simulink model "controllo_giunti_R2020b"  (R2020b)
settings: Solver=FixedStepAuto  StartTime=0.0  StopTime=1  FixedStep=0.001  RelTol=1e-3
undefined symbols (not defined in the file or in its folder): f_G1, f_G2, f_G3, f_M11, f_M12, f_M13, f_M21, f_M22, f_M23, f_M31, f_M32, f_M33, f_V1, f_V2, f_V3
libraries: robotcorelib x1
settings Model: Creator=frasi  LastModifiedBy=frasi

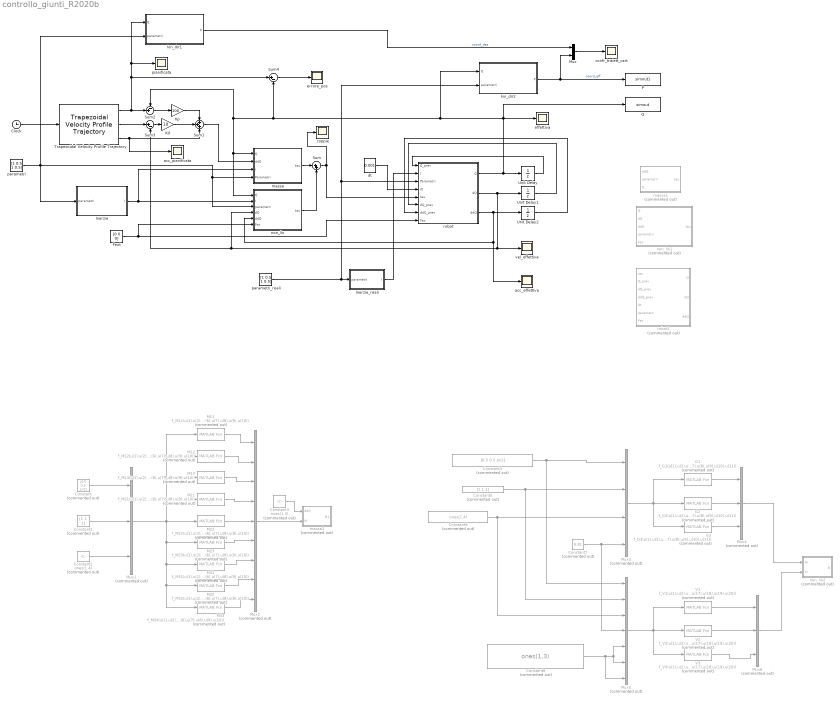
== system controllo_giunti_R2020b ==
  Clock : Clock
  Constant : Constant  Commented=on  Value=[0.5 0.5 pi/2]
  Constant1 : Constant  Commented=on  Value=[1 1 1]
  Constant2 : Constant  Commented=on  Value=ones(1,4)
  Constant3 : Constant  Commented=on  Value=ones(1,3)
  Constant4 : Constant  Commented=on  Value=[0.5 0.5 pi/2]
  Constant5 : Constant  Commented=on  Value=[1 1 1]
  Constant6 : Constant  Commented=on  Value=ones(1,4)
  Constant7 : Constant  Commented=on  Value=9.81
  Constant8 : Constant  Commented=on  Value=ones(1,3)
  Fext : Constant  Value=[0 0 0]
  G1 : MATLABFcn  Commented=on  MATLABFcn=f_G1(u(1),u(2),u(3),u(4),u(5),u(6),u(7),u(8),u(9),u(10),u(11))
  G2 : MATLABFcn  Commented=on  MATLABFcn=f_G2(u(1),u(2),u(3),u(4),u(5),u(6),u(7),u(8),u(9),u(10),u(11))
  G3 : MATLABFcn  Commented=on  MATLABFcn=f_G3(u(1),u(2),u(3),u(4),u(5),u(6),u(7),u(8),u(9),u(10),u(11))
  Inerzie : MATLAB Function  TreatAsAtomicUnit=on
  Inerzie_reali : MATLAB Function  TreatAsAtomicUnit=on
  Kd : Gain  Gain=10
  Kp : Gain  Gain=100
  M11 : MATLABFcn  Commented=on  MATLABFcn=f_M11(u(1),u(2),u(3),u(4),u(5),u(6),u(7),u(8),u(9),u(10))
  M12 : MATLABFcn  Commented=on  MATLABFcn=f_M12(u(1),u(2),u(3),u(4),u(5),u(6),u(7),u(8),u(9),u(10))
  M13 : MATLABFcn  Commented=on  MATLABFcn=f_M13(u(1),u(2),u(3),u(4),u(5),u(6),u(7),u(8),u(9),u(10))
  M21 : MATLABFcn  Commented=on  MATLABFcn=f_M21(u(1),u(2),u(3),u(4),u(5),u(6),u(7),u(8),u(9),u(10))
  M22 : MATLABFcn  Commented=on  MATLABFcn=f_M22(u(1),u(2),u(3),u(4),u(5),u(6),u(7),u(8),u(9),u(10))
  M23 : MATLABFcn  Commented=on  MATLABFcn=f_M23(u(1),u(2),u(3),u(4),u(5),u(6),u(7),u(8),u(9),u(10))
  M31 : MATLABFcn  Commented=on  MATLABFcn=f_M31(u(1),u(2),u(3),u(4),u(5),u(6),u(7),u(8),u(9),u(10))
  M32 : MATLABFcn  Commented=on  MATLABFcn=f_M32(u(1),u(2),u(3),u(4),u(5),u(6),u(7),u(8),u(9),u(10))
  M33 : MATLABFcn  Commented=on  MATLABFcn=f_M33(u(1),u(2),u(3),u(4),u(5),u(6),u(7),u(8),u(9),u(10))
  Mux : Mux  Inputs=2
  Mux1 : Mux  Commented=on  Inputs=3
  Mux2 : Mux  Commented=on  Inputs=9
  Mux3 : Mux  Commented=on
  Mux4 : Mux  Commented=on  Inputs=3
  Mux5 : Mux  Commented=on  Inputs=7
  Mux6 : Mux  Commented=on  Inputs=3
  P : ToWorkspace  VariableName=simout1  SaveFormat=Timeseries  SampleTime=-1
  Q : ToWorkspace  VariableName=simout  SaveFormat=Timeseries  SampleTime=-1
  Sum : Sum  Inputs=|++
  Sum1 : Sum  Inputs=+++
  Sum2 : Sum  Inputs=-+|
  Sum3 : Sum  Inputs=|+-
  Sum4 : Sum  Inputs=|+-
  Trapezoidal Velocity Profile Trajectory : robotcorelib/Trapezoidal Velocity Profile Trajectory  WaypointSource=Internal  Waypoints=[0.5 0.7; 0.7 0.5; pi/4 pi/3]  NumParams=1  Parameter1=End Time  Parameter2=End Time  ParameterSource=Internal  PeakVelocity=[ 2; 2 ]  Acceleration=[ 1; 2 ]  EndTime=[ 1; 1 ;1]  AccelTime=[ 1; 2 ]  SimulateUsing=Interpreted execution
      settings: SourceProductBaseCode=NV,RO,RR,UV
  Unit Delay : UnitDelay  InitialCondition=[0.5 0.7 pi/4]  SampleTime=-1  HasFrameUpgradeWarning=on
  Unit Delay1 : UnitDelay  InitialCondition=[0 0 0]  SampleTime=-1  HasFrameUpgradeWarning=on
  Unit Delay2 : UnitDelay  InitialCondition=[0 0 0]  SampleTime=-1  HasFrameUpgradeWarning=on
  V1 : MATLABFcn  Commented=on  MATLABFcn=f_V1(u(1),u(2),u(3),u(4),u(5),u(6),u(7),u(8),u(9),u(10),u(11),u(12),u(13),u(14),u(15),u(16),u(17),u(18),u(19),u(20))
  V2 : MATLABFcn  Commented=on  MATLABFcn=f_V2(u(1),u(2),u(3),u(4),u(5),u(6),u(7),u(8),u(9),u(10),u(11),u(12),u(13),u(14),u(15),u(16),u(17),u(18),u(19),u(20))
  V3 : MATLABFcn  Commented=on  MATLABFcn=f_V3(u(1),u(2),u(3),u(4),u(5),u(6),u(7),u(8),u(9),u(10),u(11),u(12),u(13),u(14),u(15),u(16),u(17),u(18),u(19),u(20))
  acc_effettiva : Scope
  acc_pianificata : Scope
  confr_traiett_cart : Scope
  coppie : Scope
  dt : Constant  Value=0.001
  effettiva : Scope
  errore_pos : Scope
  kin_dir1 : MATLAB Function  TreatAsAtomicUnit=on
  kin_dir2 : MATLAB Function  TreatAsAtomicUnit=on
  massa : Subsystem
  massa1 : MATLAB Function  Commented=on  TreatAsAtomicUnit=on
  massa2 : MATLAB Function  Commented=on  TreatAsAtomicUnit=on
  non_lin : Subsystem
  non_lin1 : MATLAB Function  Commented=on  TreatAsAtomicUnit=on
  non_lin2 : MATLAB Function  Commented=on  TreatAsAtomicUnit=on
  parametri : Constant  Value=[1 0.5 1 0.5]
  parametri_reali : Constant  Value=[1 0.5 1 0.5]
  pianificata : Scope
  robot : Subsystem
  robot1 : MATLAB Function  Commented=on  TreatAsAtomicUnit=on
  vel_effettiva : Scope
  wires:
  Clock/1 -> Trapezoidal Velocity Profile Trajectory/1
  parametri/1 -> Inerzie/1(parametri), kin_dir1/2(parametri), non_lin/3(parametri), massa/4(Parametri)
  massa/1(tau) -> Sum/1
  dt/1 -> robot/4(dt)
  robot/1(Q) -> Q/1, Sum4/2, Sum2/1, non_lin/1(Q), massa/1(Q), kin_dir2/1(Q), effettiva/1, Unit Delay/1
  robot/2(dQ) -> Unit Delay1/1, non_lin/4(dQ), Sum3/2, vel_effettiva/1
  Unit Delay/1 -> robot/1(Q_prev)
  Unit Delay1/1 -> robot/6(dQ_prev)
  Sum/1 -> robot/5(tau), coppie/1
  Trapezoidal Velocity Profile Trajectory/2 -> Sum3/1
  Sum2/1 -> Kp/1
  Sum3/1 -> Kd/1
  Kp/1 -> Sum1/1
  Kd/1 -> Sum1/2
  Trapezoidal Velocity Profile Trajectory/3 -> acc_pianificata/1, Sum1/3
  non_lin/1(tau) -> Sum/2
  Trapezoidal Velocity Profile Trajectory/1 -> Sum4/1, kin_dir1/1(Q), pianificata/1, Sum2/2
  robot/3(ddQ) -> Unit Delay2/1, acc_effettiva/1, non_lin/5(ddQ)
  parametri_reali/1 -> robot/3(Parametri), kin_dir2/2(parametri), Inerzie_reali/1(parametri)
  Sum4/1 -> errore_pos/1
  kin_dir1/1(P) -> Mux/1  "coord_des"
  kin_dir2/1(P) -> P/1, Mux/2  "coord_eff"
  Mux/1 -> confr_traiett_cart/1
  Fext/1 -> robot/8(Fex), non_lin/6(Fex)
  Sum1/1 -> massa/2(ddQ)
  Inerzie/1(I) -> massa/3(I), non_lin/2(I)
  Unit Delay2/1 -> robot/7(ddQ_prev)
  Inerzie_reali/1(I) -> robot/2(I)
  Constant2/1 -> Mux1/3
  Constant1/1 -> Mux1/2
  Constant3/1 -> massa2/1(ddQ)
  Mux1/1 -> M13/1, M12/1, M11/1, M21/1, M31/1, M32/1, M33/1, M23/1, M22/1
  M23/1 -> Mux2/6
  M33/1 -> Mux2/9
  M22/1 -> Mux2/5
  Mux2/1 -> massa2/2(M)
  M11/1 -> Mux2/1
  M32/1 -> Mux2/8
  M21/1 -> Mux2/4
  M31/1 -> Mux2/7
  Constant/1 -> Mux1/1
  M13/1 -> Mux2/3
  M12/1 -> Mux2/2
  Constant6/1 -> Mux3/3, Mux5/3
  Constant5/1 -> Mux5/2, Mux3/2
  Mux4/1 -> non_lin2/1(Gi)
  Mux5/1 -> V3/1, V2/1, V1/1
  Constant8/1 -> Mux5/7, Mux5/5, Mux5/6
  G2/1 -> Mux4/2
  Constant7/1 -> Mux5/4, Mux3/4
  Constant4/1 -> Mux5/1, Mux3/1
  Mux3/1 -> G3/1, G2/1, G1/1
  G1/1 -> Mux4/1
  G3/1 -> Mux4/3
  V1/1 -> Mux6/1
  V2/1 -> Mux6/2
  V3/1 -> Mux6/3
  Mux6/1 -> non_lin2/2(Vi)

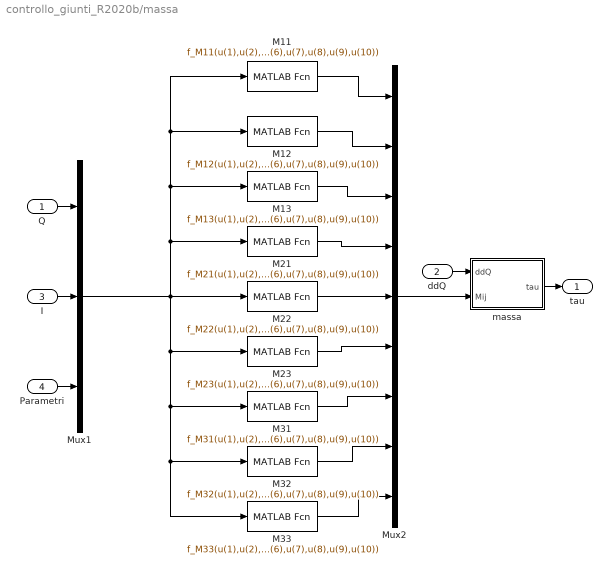
== system controllo_giunti_R2020b/massa ==
  Q : Inport
  ddQ : Inport  Port=2
  I : Inport  Port=3
  Parametri : Inport  Port=4
  M11 : MATLABFcn  MATLABFcn=f_M11(u(1),u(2),u(3),u(4),u(5),u(6),u(7),u(8),u(9),u(10))
  M12 : MATLABFcn  MATLABFcn=f_M12(u(1),u(2),u(3),u(4),u(5),u(6),u(7),u(8),u(9),u(10))
  M13 : MATLABFcn  MATLABFcn=f_M13(u(1),u(2),u(3),u(4),u(5),u(6),u(7),u(8),u(9),u(10))
  M21 : MATLABFcn  MATLABFcn=f_M21(u(1),u(2),u(3),u(4),u(5),u(6),u(7),u(8),u(9),u(10))
  M22 : MATLABFcn  MATLABFcn=f_M22(u(1),u(2),u(3),u(4),u(5),u(6),u(7),u(8),u(9),u(10))
  M23 : MATLABFcn  MATLABFcn=f_M23(u(1),u(2),u(3),u(4),u(5),u(6),u(7),u(8),u(9),u(10))
  M31 : MATLABFcn  MATLABFcn=f_M31(u(1),u(2),u(3),u(4),u(5),u(6),u(7),u(8),u(9),u(10))
  M32 : MATLABFcn  MATLABFcn=f_M32(u(1),u(2),u(3),u(4),u(5),u(6),u(7),u(8),u(9),u(10))
  M33 : MATLABFcn  MATLABFcn=f_M33(u(1),u(2),u(3),u(4),u(5),u(6),u(7),u(8),u(9),u(10))
  Mux1 : Mux  Inputs=3
  Mux2 : Mux  Inputs=9
  massa : MATLAB Function  TreatAsAtomicUnit=on
  tau : Outport
  wires:
  M13/1 -> Mux2/3
  Mux2/1 -> massa/2(Mij)
  M33/1 -> Mux2/9
  M11/1 -> Mux2/1
  Mux1/1 -> M13/1, M12/1, M11/1, M21/1, M31/1, M32/1, M33/1, M23/1, M22/1
  M22/1 -> Mux2/5
  M23/1 -> Mux2/6
  M31/1 -> Mux2/7
  M21/1 -> Mux2/4
  M12/1 -> Mux2/2
  Parametri/1 -> Mux1/3
  M32/1 -> Mux2/8
  ddQ/1 -> massa/1(ddQ)
  I/1 -> Mux1/2
  Q/1 -> Mux1/1
  massa/1(tau) -> tau/1

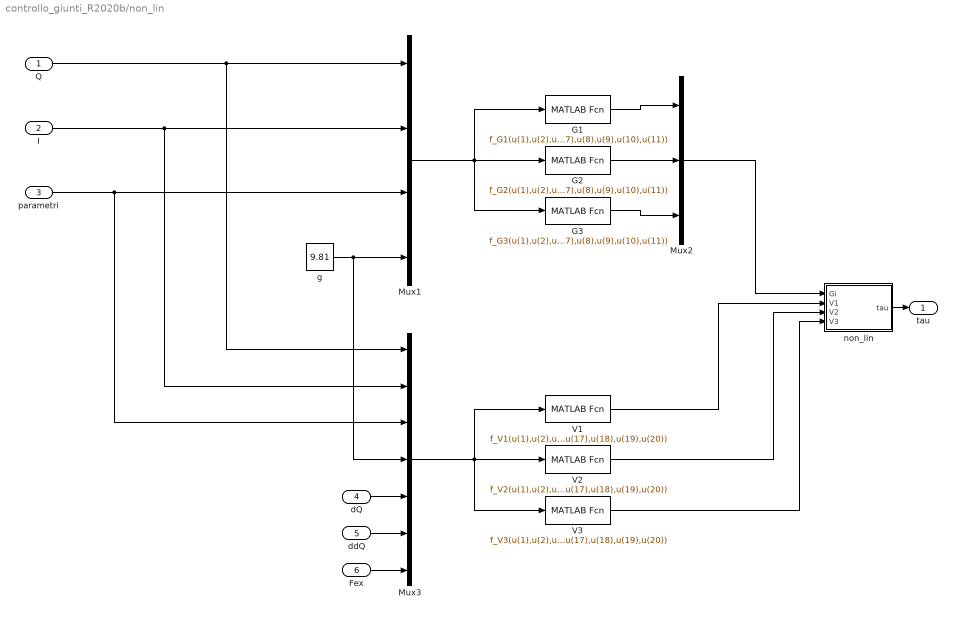
== system controllo_giunti_R2020b/non_lin ==
  Q : Inport
  I : Inport  Port=2
  parametri : Inport  Port=3
  dQ : Inport  Port=4
  ddQ : Inport  Port=5
  Fex : Inport  Port=6
  G1 : MATLABFcn  MATLABFcn=f_G1(u(1),u(2),u(3),u(4),u(5),u(6),u(7),u(8),u(9),u(10),u(11))
  G2 : MATLABFcn  MATLABFcn=f_G2(u(1),u(2),u(3),u(4),u(5),u(6),u(7),u(8),u(9),u(10),u(11))
  G3 : MATLABFcn  MATLABFcn=f_G3(u(1),u(2),u(3),u(4),u(5),u(6),u(7),u(8),u(9),u(10),u(11))
  Mux1 : Mux
  Mux2 : Mux  Inputs=3
  Mux3 : Mux  Inputs=7
  V1 : MATLABFcn  MATLABFcn=f_V1(u(1),u(2),u(3),u(4),u(5),u(6),u(7),u(8),u(9),u(10),u(11),u(12),u(13),u(14),u(15),u(16),u(17),u(18),u(19),u(20))
  V2 : MATLABFcn  MATLABFcn=f_V2(u(1),u(2),u(3),u(4),u(5),u(6),u(7),u(8),u(9),u(10),u(11),u(12),u(13),u(14),u(15),u(16),u(17),u(18),u(19),u(20))
  V3 : MATLABFcn  MATLABFcn=f_V3(u(1),u(2),u(3),u(4),u(5),u(6),u(7),u(8),u(9),u(10),u(11),u(12),u(13),u(14),u(15),u(16),u(17),u(18),u(19),u(20))
  g : Constant  Value=9.81
  non_lin : MATLAB Function  TreatAsAtomicUnit=on
  tau : Outport
  wires:
  Mux3/1 -> V3/1, V2/1, V1/1
  g/1 -> Mux3/4, Mux1/4
  G2/1 -> Mux2/2
  parametri/1 -> Mux3/3, Mux1/3
  Mux1/1 -> G3/1, G2/1, G1/1
  G1/1 -> Mux2/1
  G3/1 -> Mux2/3
  non_lin/1(tau) -> tau/1
  Mux2/1 -> non_lin/1(Gi)
  Q/1 -> Mux3/1, Mux1/1
  Fex/1 -> Mux3/7
  I/1 -> Mux3/2, Mux1/2
  dQ/1 -> Mux3/5
  ddQ/1 -> Mux3/6
  V1/1 -> non_lin/2(V1)
  V2/1 -> non_lin/3(V2)
  V3/1 -> non_lin/4(V3)

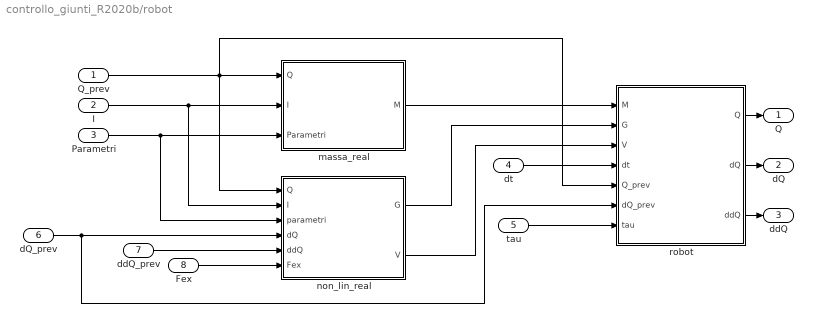
== system controllo_giunti_R2020b/robot ==
  Q_prev : Inport
  I : Inport  Port=2
  Parametri : Inport  Port=3
  dt : Inport  Port=4
  tau : Inport  Port=5
  dQ_prev : Inport  Port=6
  ddQ_prev : Inport  Port=7
  Fex : Inport  Port=8
  massa_real : Subsystem
  non_lin_real : Subsystem
  robot : MATLAB Function  TreatAsAtomicUnit=on
  Q : Outport
  dQ : Outport  Port=2
  ddQ : Outport  Port=3
  wires:
  Parametri/1 -> non_lin_real/3(parametri), massa_real/3(Parametri)
  non_lin_real/1(G) -> robot/2(G)
  ddQ_prev/1 -> non_lin_real/5(ddQ)
  Fex/1 -> non_lin_real/6(Fex)
  non_lin_real/2(V) -> robot/3(V)
  I/1 -> non_lin_real/2(I), massa_real/2(I)
  massa_real/1(M) -> robot/1(M)
  robot/1(Q) -> Q/1
  Q_prev/1 -> robot/5(Q_prev), massa_real/1(Q), non_lin_real/1(Q)
  dQ_prev/1 -> robot/6(dQ_prev), non_lin_real/4(dQ)
  tau/1 -> robot/7(tau)
  robot/2(dQ) -> dQ/1
  dt/1 -> robot/4(dt)
  robot/3(ddQ) -> ddQ/1

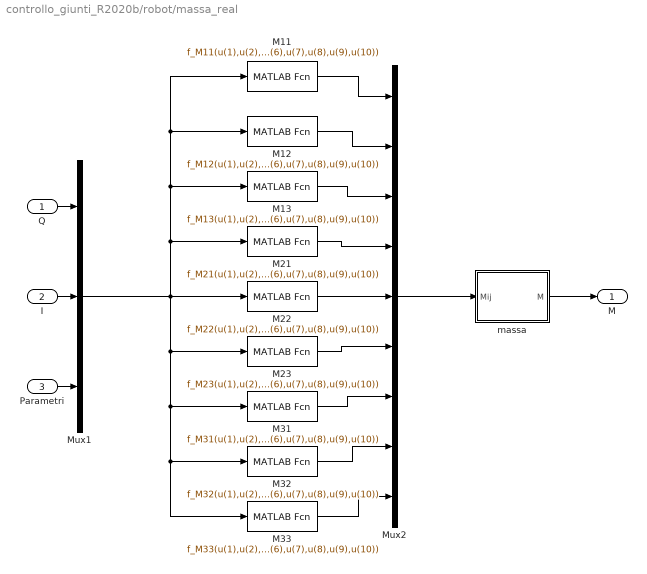
== system controllo_giunti_R2020b/robot/massa_real ==
  Q : Inport
  I : Inport  Port=2
  Parametri : Inport  Port=3
  M11 : MATLABFcn  MATLABFcn=f_M11(u(1),u(2),u(3),u(4),u(5),u(6),u(7),u(8),u(9),u(10))
  M12 : MATLABFcn  MATLABFcn=f_M12(u(1),u(2),u(3),u(4),u(5),u(6),u(7),u(8),u(9),u(10))
  M13 : MATLABFcn  MATLABFcn=f_M13(u(1),u(2),u(3),u(4),u(5),u(6),u(7),u(8),u(9),u(10))
  M21 : MATLABFcn  MATLABFcn=f_M21(u(1),u(2),u(3),u(4),u(5),u(6),u(7),u(8),u(9),u(10))
  M22 : MATLABFcn  MATLABFcn=f_M22(u(1),u(2),u(3),u(4),u(5),u(6),u(7),u(8),u(9),u(10))
  M23 : MATLABFcn  MATLABFcn=f_M23(u(1),u(2),u(3),u(4),u(5),u(6),u(7),u(8),u(9),u(10))
  M31 : MATLABFcn  MATLABFcn=f_M31(u(1),u(2),u(3),u(4),u(5),u(6),u(7),u(8),u(9),u(10))
  M32 : MATLABFcn  MATLABFcn=f_M32(u(1),u(2),u(3),u(4),u(5),u(6),u(7),u(8),u(9),u(10))
  M33 : MATLABFcn  MATLABFcn=f_M33(u(1),u(2),u(3),u(4),u(5),u(6),u(7),u(8),u(9),u(10))
  Mux1 : Mux  Inputs=3
  Mux2 : Mux  Inputs=9
  massa : MATLAB Function  TreatAsAtomicUnit=on
  M : Outport
  wires:
  M13/1 -> Mux2/3
  Mux2/1 -> massa/1(Mij)
  M33/1 -> Mux2/9
  M11/1 -> Mux2/1
  Mux1/1 -> M13/1, M12/1, M11/1, M21/1, M31/1, M32/1, M33/1, M23/1, M22/1
  M22/1 -> Mux2/5
  M23/1 -> Mux2/6
  M31/1 -> Mux2/7
  M21/1 -> Mux2/4
  M12/1 -> Mux2/2
  Parametri/1 -> Mux1/3
  M32/1 -> Mux2/8
  I/1 -> Mux1/2
  Q/1 -> Mux1/1
  massa/1(M) -> M/1

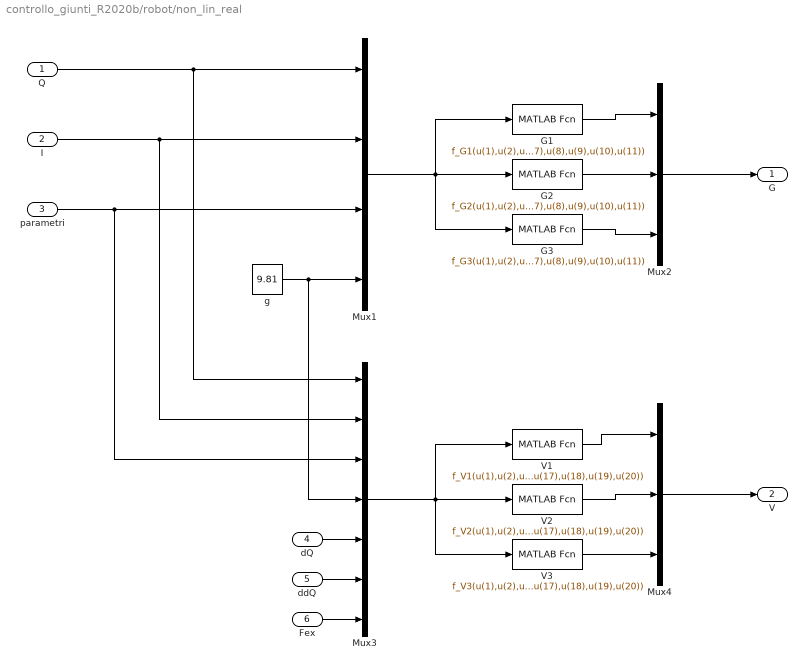
== system controllo_giunti_R2020b/robot/non_lin_real ==
  Q : Inport
  I : Inport  Port=2
  parametri : Inport  Port=3
  dQ : Inport  Port=4
  ddQ : Inport  Port=5
  Fex : Inport  Port=6
  G1 : MATLABFcn  MATLABFcn=f_G1(u(1),u(2),u(3),u(4),u(5),u(6),u(7),u(8),u(9),u(10),u(11))
  G2 : MATLABFcn  MATLABFcn=f_G2(u(1),u(2),u(3),u(4),u(5),u(6),u(7),u(8),u(9),u(10),u(11))
  G3 : MATLABFcn  MATLABFcn=f_G3(u(1),u(2),u(3),u(4),u(5),u(6),u(7),u(8),u(9),u(10),u(11))
  Mux1 : Mux
  Mux2 : Mux  Inputs=3
  Mux3 : Mux  Inputs=7
  Mux4 : Mux  Inputs=3
  V1 : MATLABFcn  MATLABFcn=f_V1(u(1),u(2),u(3),u(4),u(5),u(6),u(7),u(8),u(9),u(10),u(11),u(12),u(13),u(14),u(15),u(16),u(17),u(18),u(19),u(20))
  V2 : MATLABFcn  MATLABFcn=f_V2(u(1),u(2),u(3),u(4),u(5),u(6),u(7),u(8),u(9),u(10),u(11),u(12),u(13),u(14),u(15),u(16),u(17),u(18),u(19),u(20))
  V3 : MATLABFcn  MATLABFcn=f_V3(u(1),u(2),u(3),u(4),u(5),u(6),u(7),u(8),u(9),u(10),u(11),u(12),u(13),u(14),u(15),u(16),u(17),u(18),u(19),u(20))
  g : Constant  Value=9.81
  G : Outport
  V : Outport  Port=2
  wires:
  Mux3/1 -> V3/1, V2/1, V1/1
  g/1 -> Mux3/4, Mux1/4
  V2/1 -> Mux4/2
  G2/1 -> Mux2/2
  Q/1 -> Mux3/1, Mux1/1
  Mux1/1 -> G3/1, G2/1, G1/1
  V3/1 -> Mux4/3
  V1/1 -> Mux4/1
  G1/1 -> Mux2/1
  G3/1 -> Mux2/3
  Mux4/1 -> V/1
  Mux2/1 -> G/1
  parametri/1 -> Mux3/3, Mux1/3
  Fex/1 -> Mux3/7
  I/1 -> Mux3/2, Mux1/2
  ddQ/1 -> Mux3/6
  dQ/1 -> Mux3/5

== matlab function controllo_giunti_R2020b/robot/robot ==
  data: M input; Q output; G input; V input; dt input; Q_prev input; dQ_prev input; dQ output; ddQ output; tau input
function [Q,dQ,ddQ] = robot(M,G,V,dt,Q_prev,dQ_prev,tau)
%ddq=inv(M)*(tau-N)  (N=V+G)
ddQ=M\(tau-V-G);
dQ=dQ_prev+ddQ*dt;
Q=Q_prev+dQ*dt;
end

== matlab function controllo_giunti_R2020b/Inerzie_reali ==
  data: parametri input; I output
function I = Inerzie(parametri)
l=parametri(1);
d=parametri(2);
%m1=parametri(3);
ma=parametri(4);


I2 = ma*l^2/4 + 1/12 *ma*l^2;
I5 = I2;
I3 = I2 + 1/12 * ma*d^2 + ma*(d^2/4+l^2/4);
I=[I2;I5;I3];
end

== matlab function controllo_giunti_R2020b/massa2 ==
  data: ddQ input; M input; M1 output
function M1 = massa(ddQ,M)

M1=[M(1) M(2) M(3);M(4) M(5) M(6);M(7) M(8) M(9)]

end

== matlab function controllo_giunti_R2020b/non_lin2 ==
  data: Gi input; N output; Vi input
function N   = non_lin(Gi,Vi)

G=[Gi(1);Gi(2);Gi(3)];
V=[Vi(1);Vi(2);Vi(3)];

N = (G + V);

end

== matlab function controllo_giunti_R2020b/non_lin1 ==
  data: Q input; tau output; dQ input; ddQ input; parametri input; Fex input
function tau = non_lin(Q,dQ,ddQ,parametri,Fex)
l=parametri(1);
d=parametri(2);
m1=parametri(3);
ma=parametri(4);

xc1=Q(1);
xc5=Q(2);
q2=Q(3);

dxc1=dQ(1);
dxc5=dQ(2);
dq2=dQ(3);

ddxc1=ddQ(1);
ddxc5=ddQ(2);
ddq2=ddQ(3);

Fx=Fex(1);
Fy=Fex(2);
Mf=Fex(3);

I2 = ma*l^2/4 + 1/12 *ma*l^2;
I5 = I2;
I3 = I2 + 1/12 * ma*d^2 + ma*(d^2/4+l^2/4);

G1=f_G1(xc1,xc5,q2,I2,I5,I3,l,d,m1,ma);
G2=f_G2(xc1,xc5,q2,I2,I5,I3,l,d,m1,ma);
G3=f_G3(xc1,xc5,q2,I2,I5,I3,l,d,m1,ma);
G=[G1;G2;G3];

V1=f_V1(xc1,xc5,q2,I2,I5,I3,l,d,m1,ma,dxc1,dxc5,dq2,ddxc1,ddxc5,ddq2,Fx,Fy,Mf);
V2=f_V2(xc1,xc5,q2,I2,I5,I3,l,d,m1,ma,dxc1,dxc5,dq2,ddxc1,ddxc5,ddq2,Fx,Fy,Mf);
V3=f_V3(xc1,xc5,q2,I2,I5,I3,l,d,m1,ma,dxc1,dxc5,dq2,ddxc1,ddxc5,ddq2,Fx,Fy,Mf);
V=[V1;V2;V3];

N=G+V;

tau=N;
end

== matlab function controllo_giunti_R2020b/non_lin/non_lin ==
  data: Gi input; tau output; V1 input; V2 input; V3 input
function tau = non_lin(Gi,V1,V2,V3)

G=[Gi(1);Gi(2);Gi(3)];
V=[V1;V2;V3];

tau=G+V;
end

== matlab function controllo_giunti_R2020b/robot1 ==
  data: tau input; Q output; Q_prev input; dQ_prev input; ddQ_prev input; dt input; parametri input; dQ output; ddQ output; Fex input
function [Q,dQ,ddQ] = robot(tau,Q_prev,dQ_prev,ddQ_prev,dt,parametri,Fex)%conosco tau e devo calcolare la velocità, è un problema di dinamica diretta
xc1=Q_prev(1);
xc5=Q_prev(2);
q2=Q_prev(3);

dxc1=dQ_prev(1);
dxc5=dQ_prev(2);
dq2=dQ_prev(3);

ddxc1=ddQ_prev(1);
ddxc5=ddQ_prev(2);
ddq2=ddQ_prev(3);

l=parametri(1);
d=parametri(2);
m1=parametri(3);
ma=parametri(4);
g=9.81;

Fx=Fex(1);
Fy=Fex(2);
Mf=Fex(3);

I2 = ma*l^2/4 + 1/12 *ma*l^2;
I5 = I2;
I3 = I2 + 1/12 * ma*d^2 + ma*(d^2/4+l^2/4);

M11=f_M11(xc1,xc5,q2,I2,I5,I3,l,d,m1,ma);
M12=f_M12(xc1,xc5,q2,I2,I5,I3,l,d,m1,ma);
M13=f_M13(xc1,xc5,q2,I2,I5,I3,l,d,m1,ma);
M21=f_M21(xc1,xc5,q2,I2,I5,I3,l,d,m1,ma);
M22=f_M22(xc1,xc5,q2,I2,I5,I3,l,d,m1,ma);
M23=f_M23(xc1,xc5,q2,I2,I5,I3,l,d,m1,ma);
M31=f_M31(xc1,xc5,q2,I2,I5,I3,l,d,m1,ma);
M32=f_M32(xc1,xc5,q2,I2,I5,I3,l,d,m1,ma);
M33=f_M33(xc1,xc5,q2,I2,I5,I3,l,d,m1,ma);
M=[M11 M12 M13;M21 M22 M23;M31 M32 M33];

G1=f_G1(xc1,xc5,q2,I2,I5,I3,l,d,m1,ma);
G2=f_G2(xc1,xc5,q2,I2,I5,I3,l,d,m1,ma);
G3=f_G3(xc1,xc5,q2,I2,I5,I3,l,d,m1,ma);
G=[G1;G2;G3];

V1=f_V1(xc1,xc5,q2,I2,I5,I3,l,d,m1,ma,dxc1,dxc5,dq2,ddxc1,ddxc5,ddq2,Fx,Fy,Mf);
V2=f_V2(xc1,xc5,q2,I2,I5,I3,l,d,m1,ma,dxc1,dxc5,dq2,ddxc1,ddxc5,ddq2,Fx,Fy,Mf);
V3=f_V3(xc1,xc5,q2,I2,I5,I3,l,d,m1,ma,dxc1,dxc5,dq2,ddxc1,ddxc5,ddq2,Fx,Fy,Mf);
V=[V1;V2;V3];

%ddq=inv(M)*(tau-N)  (N=V+G)
ddQ=M\(tau-V-G);
dQ=dQ_prev+ddQ*dt;
Q=Q_prev+dQ*dt;
end

== matlab function controllo_giunti_R2020b/kin_dir1 ==
  data: Q input; P output; parametri input
function P  = kin_dir_pos(Q,parametri) %P[X Y alpha]
l=parametri(1);
d=parametri(2);
m1=parametri(3);
ma=parametri(4);
xc1=Q(1);
xc5=Q(2);
q2=Q(3);


q3 = ...
 -q2 - 2*atan((2*l*xc5 + (-(2*l*xc1 + l^2 + l^2*tan(q2/2)^2 + xc1^2 + xc5^2 + xc1^2*tan(q2/2)^2 + xc5^2*tan(q2/2)^2 - 4*l*xc5*tan(q2/2) - 2*l*xc1*tan(q2/2)^2)*(2*l*xc1 - 3*l^2 - 3*l^2*tan(q2/2)^2 + xc1^2 + xc5^2 + xc1^2*tan(q2/2)^2 + xc5^2*tan(q2/2)^2 - 4*l*xc5*tan(q2/2) - 2*l*xc1*tan(q2/2)^2))^(1/2) - 4*l^2*tan(q2/2) + 2*l*xc5*tan(q2/2)^2)/(3*l^2*tan(q2/2)^2 - l^2 + xc1^2 + xc5^2 + xc1^2*tan(q2/2)^2 + xc5^2*tan(q2/2)^2 - 4*l*xc5*tan(q2/2) - 4*l*xc1*tan(q2/2)^2) - (4*(l*xc5 - 2*l^2*tan(q2/2) + l*xc5*tan(q2/2)^2))/(3*l^2*tan(q2/2)^2 - l^2 + xc1^2 + xc5^2 + xc1^2*tan(q2/2)^2 + xc5^2*tan(q2/2)^2 - 4*l*xc5*tan(q2/2) - 4*l*xc1*tan(q2/2)^2));
q4 = ...
2*atan((2*l*xc5 + (-(2*l*xc1 + l^2 + l^2*tan(q2/2)^2 + xc1^2 + xc5^2 + xc1^2*tan(q2/2)^2 + xc5^2*tan(q2/2)^2 - 4*l*xc5*tan(q2/2) - 2*l*xc1*tan(q2/2)^2)*(2*l*xc1 - 3*l^2 - 3*l^2*tan(q2/2)^2 + xc1^2 + xc5^2 + xc1^2*tan(q2/2)^2 + xc5^2*tan(q2/2)^2 - 4*l*xc5*tan(q2/2) - 2*l*xc1*tan(q2/2)^2))^(1/2) - 4*l^2*tan(q2/2) + 2*l*xc5*tan(q2/2)^2)/(3*l^2*tan(q2/2)^2 - l^2 + xc1^2 + xc5^2 + xc1^2*tan(q2/2)^2 + xc5^2*tan(q2/2)^2 - 4*l*xc5*tan(q2/2) - 4*l*xc1*tan(q2/2)^2)) + 2*atan((2*l*xc5 + (-(2*l*xc1 + l^2 + l^2*tan(q2/2)^2 + xc1^2 + xc5^2 + xc1^2*tan(q2/2)^2 + xc5^2*tan(q2/2)^2 - 4*l*xc5*tan(q2/2) - 2*l*xc1*tan(q2/2)^2)*(2*l*xc1 - 3*l^2 - 3*l^2*tan(q2/2)^2 + xc1^2 + xc5^2 + xc1^2*tan(q2/2)^2 + xc5^2*tan(q2/2)^2 - 4*l*xc5*tan(q2/2) - 2*l*xc1*tan(q2/2)^2))^(1/2) - 4*l^2*tan(q2/2) + 2*l*xc5*tan(q2/2)^2)/(3*l^2*tan(q2/2)^2 - l^2 + xc1^2 + xc5^2 + xc1^2*tan(q2/2)^2 + xc5^2*tan(q2/2)^2 - 4*l*xc5*tan(q2/2) - 4*l*xc1*tan(q2/2)^2) - (4*(l*xc5 - 2*l^2*tan(q2/2) + l*xc5*tan(q2/2)^2))/(3*l^2*tan(q2/2)^2 - l^2 + xc1^2 + xc5^2 + xc1^2*tan(q2/2)^2 + xc5^2*tan(q2/2)^2 - 4*l*xc5*tan(q2/2) - 4*l*xc1*tan(q2/2)^2));


gamma = q2+q3;
%beta = q2+q3+q4;
alpha=gamma-pi/2;

P=zeros(3,1);
P(1) = xc1+l*cos(q2)+l/2*cos(gamma)+d*cos(alpha);
P(2) = l*sin(q2)+l/2*sin(gamma)+d*sin(alpha);
P(3) = q2 + q3 - pi/2;

end

== matlab function controllo_giunti_R2020b/kin_dir2 ==
  data: Q input; P output; parametri input
function P  = kin_dir_pos(Q,parametri) %P[X Y alpha]
l=parametri(1);
d=parametri(2);
m1=parametri(3);
ma=parametri(4);
xc1=Q(1);
xc5=Q(2);
q2=Q(3);


q3 = ...
 -q2 - 2*atan((2*l*xc5 + (-(2*l*xc1 + l^2 + l^2*tan(q2/2)^2 + xc1^2 + xc5^2 + xc1^2*tan(q2/2)^2 + xc5^2*tan(q2/2)^2 - 4*l*xc5*tan(q2/2) - 2*l*xc1*tan(q2/2)^2)*(2*l*xc1 - 3*l^2 - 3*l^2*tan(q2/2)^2 + xc1^2 + xc5^2 + xc1^2*tan(q2/2)^2 + xc5^2*tan(q2/2)^2 - 4*l*xc5*tan(q2/2) - 2*l*xc1*tan(q2/2)^2))^(1/2) - 4*l^2*tan(q2/2) + 2*l*xc5*tan(q2/2)^2)/(3*l^2*tan(q2/2)^2 - l^2 + xc1^2 + xc5^2 + xc1^2*tan(q2/2)^2 + xc5^2*tan(q2/2)^2 - 4*l*xc5*tan(q2/2) - 4*l*xc1*tan(q2/2)^2) - (4*(l*xc5 - 2*l^2*tan(q2/2) + l*xc5*tan(q2/2)^2))/(3*l^2*tan(q2/2)^2 - l^2 + xc1^2 + xc5^2 + xc1^2*tan(q2/2)^2 + xc5^2*tan(q2/2)^2 - 4*l*xc5*tan(q2/2) - 4*l*xc1*tan(q2/2)^2));
q4 = ...
2*atan((2*l*xc5 + (-(2*l*xc1 + l^2 + l^2*tan(q2/2)^2 + xc1^2 + xc5^2 + xc1^2*tan(q2/2)^2 + xc5^2*tan(q2/2)^2 - 4*l*xc5*tan(q2/2) - 2*l*xc1*tan(q2/2)^2)*(2*l*xc1 - 3*l^2 - 3*l^2*tan(q2/2)^2 + xc1^2 + xc5^2 + xc1^2*tan(q2/2)^2 + xc5^2*tan(q2/2)^2 - 4*l*xc5*tan(q2/2) - 2*l*xc1*tan(q2/2)^2))^(1/2) - 4*l^2*tan(q2/2) + 2*l*xc5*tan(q2/2)^2)/(3*l^2*tan(q2/2)^2 - l^2 + xc1^2 + xc5^2 + xc1^2*tan(q2/2)^2 + xc5^2*tan(q2/2)^2 - 4*l*xc5*tan(q2/2) - 4*l*xc1*tan(q2/2)^2)) + 2*atan((2*l*xc5 + (-(2*l*xc1 + l^2 + l^2*tan(q2/2)^2 + xc1^2 + xc5^2 + xc1^2*tan(q2/2)^2 + xc5^2*tan(q2/2)^2 - 4*l*xc5*tan(q2/2) - 2*l*xc1*tan(q2/2)^2)*(2*l*xc1 - 3*l^2 - 3*l^2*tan(q2/2)^2 + xc1^2 + xc5^2 + xc1^2*tan(q2/2)^2 + xc5^2*tan(q2/2)^2 - 4*l*xc5*tan(q2/2) - 2*l*xc1*tan(q2/2)^2))^(1/2) - 4*l^2*tan(q2/2) + 2*l*xc5*tan(q2/2)^2)/(3*l^2*tan(q2/2)^2 - l^2 + xc1^2 + xc5^2 + xc1^2*tan(q2/2)^2 + xc5^2*tan(q2/2)^2 - 4*l*xc5*tan(q2/2) - 4*l*xc1*tan(q2/2)^2) - (4*(l*xc5 - 2*l^2*tan(q2/2) + l*xc5*tan(q2/2)^2))/(3*l^2*tan(q2/2)^2 - l^2 + xc1^2 + xc5^2 + xc1^2*tan(q2/2)^2 + xc5^2*tan(q2/2)^2 - 4*l*xc5*tan(q2/2) - 4*l*xc1*tan(q2/2)^2));


gamma = q2+q3;
%beta = q2+q3+q4;
alpha=gamma-pi/2;

P=zeros(3,1);
P(1) = xc1+l*cos(q2)+l/2*cos(gamma)+d*cos(alpha);
P(2) = l*sin(q2)+l/2*sin(gamma)+d*sin(alpha);
P(3) = q2 + q3 - pi/2;

end

== matlab function controllo_giunti_R2020b/massa/massa ==
  data: ddQ input; tau output; Mij input
function  tau= massa(ddQ,Mij)

M=[Mij(1) Mij(2) Mij(3);Mij(4) Mij(5) Mij(6);Mij(7) Mij(8) Mij(9)];
tau=M*ddQ;

end

== matlab function controllo_giunti_R2020b/Inerzie ==
  data: parametri input; I output
function I = Inerzie(parametri)
l=parametri(1);
d=parametri(2);
%m1=parametri(3);
ma=parametri(4);


I2 = ma*l^2/4 + 1/12 *ma*l^2;
I5 = I2;
I3 = I2 + 1/12 * ma*d^2 + ma*(d^2/4+l^2/4);
I=[I2;I5;I3];
end

== matlab function controllo_giunti_R2020b/massa1 ==
  data: ddQ input; parametri input; tau output; Q input
function tau = massa(ddQ,parametri,Q)
l=parametri(1);
d=parametri(2);
m1=parametri(3);
ma=parametri(4);

xc1=Q(1);
xc5=Q(2);
q2=Q(3);


I2 = ma*l^2/4 + 1/12 *ma*l^2;
I5 = I2;
I3 = I2 + 1/12 * ma*d^2 + ma*(d^2/4+l^2/4);

M11=f_M11(xc1,xc5,q2,I2,I5,I3,l,d,m1,ma);
M12=f_M12(xc1,xc5,q2,I2,I5,I3,l,d,m1,ma);
M13=f_M13(xc1,xc5,q2,I2,I5,I3,l,d,m1,ma);
M21=f_M21(xc1,xc5,q2,I2,I5,I3,l,d,m1,ma);
M22=f_M22(xc1,xc5,q2,I2,I5,I3,l,d,m1,ma);
M23=f_M23(xc1,xc5,q2,I2,I5,I3,l,d,m1,ma);
M31=f_M31(xc1,xc5,q2,I2,I5,I3,l,d,m1,ma);
M32=f_M32(xc1,xc5,q2,I2,I5,I3,l,d,m1,ma);
M33=f_M33(xc1,xc5,q2,I2,I5,I3,l,d,m1,ma);
M=[M11 M12 M13;M21 M22 M23;M31 M32 M33];

tau=M*ddQ;
end

== matlab function controllo_giunti_R2020b/robot/massa_real/massa ==
  data: M output; Mij input
function  M= matrice_massa(Mij)

M=[Mij(1) Mij(2) Mij(3);Mij(4) Mij(5) Mij(6);Mij(7) Mij(8) Mij(9)];

end
